simulink library "Battery"  (R2015a)
settings: Solver=ode45  StartTime=0.0  StopTime=10.0  RelTol=1e-3
undefined symbols (not defined in the file): Battery, Env, magnitude
libraries: fl_lib x10, nesl_utility x5
settings Model: Creator=tbria  LastModifiedBy=BRIAN

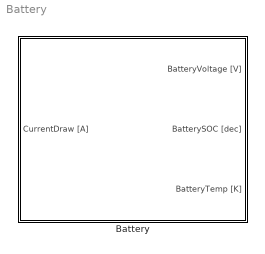
== system Battery ==
  Battery : Subsystem

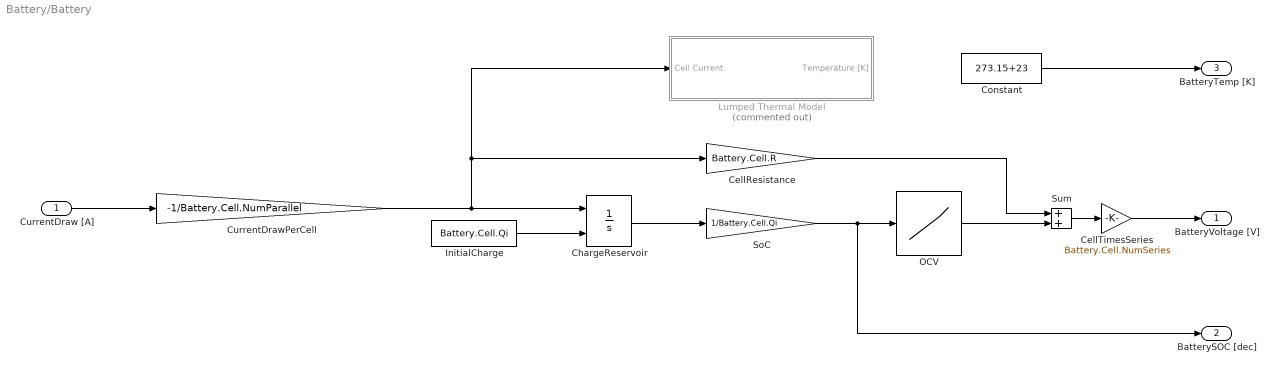
== system Battery/Battery ==
  CurrentDraw [A] : Inport
  CellResistance : Gain  Gain=Battery.Cell.R
  CellTimesSeries : Gain  Gain=Battery.Cell.NumSeries
  ChargeReservoir : Integrator  InitialConditionSource=external
  Constant : Constant  Value=273.15+23
  CurrentDrawPerCell : Gain  Gain=-1/Battery.Cell.NumParallel
  InitialCharge : Constant  Value=Battery.Cell.Qi
  Lumped Thermal Model : Subsystem  Commented=on
  OCV : Lookup_n-D  NumberOfTableDimensions=1  BreakpointsForDimension1=Battery.Cell.VoltOC.SoC  Table=Battery.Cell.VoltOC.Voltage  InternalRulePriority=Speed  RndMeth=Simplest  InputSameDT=on
  SoC : Gain  Gain=1/Battery.Cell.Qi
  Sum : Sum
  BatteryVoltage [V] : Outport
  BatterySOC [dec] : Outport  Port=2
  BatteryTemp [K] : Outport  Port=3
  wires:
  Constant/1 -> BatteryTemp [K]/1
  CurrentDraw [A]/1 -> CurrentDrawPerCell/1
  InitialCharge/1 -> ChargeReservoir/2
  ChargeReservoir/1 -> SoC/1
  SoC/1 -> OCV/1, BatterySOC [dec]/1
  CellTimesSeries/1 -> BatteryVoltage [V]/1
  CellResistance/1 -> Sum/1
  OCV/1 -> Sum/2
  Sum/1 -> CellTimesSeries/1
  CurrentDrawPerCell/1 -> Lumped Thermal Model/1(Cell Current), CellResistance/1, ChargeReservoir/1

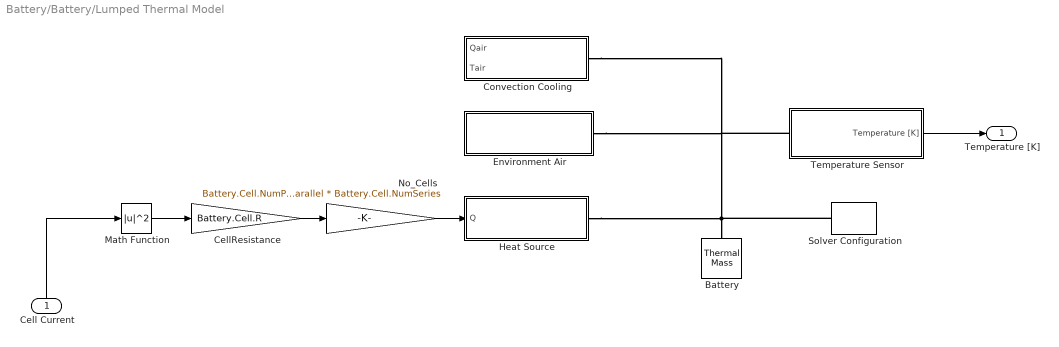
== system Battery/Battery/Lumped Thermal Model ==
  Cell Current : Inport
  Battery : fl_lib/Thermal/Thermal Elements/Thermal Mass  mass=Battery.Cell.m*Battery.Cell.NumParallel * Battery.Cell.NumSeries kg  sp_heat=Battery.Cell.c J/kg/K  Q_specify=off  Q_priority=High  Q=0 J/s  T_specify=off  T_priority=High  T=300 K
  CellResistance : Gain  Gain=Battery.Cell.R
  Convection Cooling : Subsystem
  Environment Air : Subsystem
  Heat Source : Subsystem
  Math Function : Math  Operator=magnitude^2  SaturateOnIntegerOverflow=on
  No_Cells : Gain  Gain=Battery.Cell.NumParallel * Battery.Cell.NumSeries
  Solver Configuration : nesl_utility/Solver Configuration  PhysicalDomain=network_engine_domain  SubClassName=solver  LeftPortType=input  RightPortType=generic  Accelerate=off  Tones=[]  Harmonics=[]  SimulateNoise=off  Profile=off  UseLocalSampling=off  EnableSwitchedLinearOptims=on  FrequencyDomain=off  UseCCode=off  RelTol=0.001  AbsTol=1e-06  MinStep=1e-09  ToWorkspace=off  RevertToSquareIcSolve=off  NumHomotopyIterations=100  DoDC=off  ResidualTolerance=1e-09  UseLocalSolver=off  LocalSolverChoice=NE_BACKWARD_EULER_ADVANCER  LocalSolverSampleTime=0.001  DoFixedCost=off  MaxNonlinIter=3  MaxModeIter=2  LinearAlgebra=Sparse  DelaysMemoryBudget=1024  AutomaticFiltering=on  FilteringTimeConstant=0.001
  Temperature Sensor : Subsystem
  Temperature [K] : Outport
  wires:
  Math Function/1 -> CellResistance/1
  CellResistance/1 -> No_Cells/1
  No_Cells/1 -> Heat Source/1(Q)
  Temperature Sensor/1(Temperature [K]) -> Temperature [K]/1
  Cell Current/1 -> Math Function/1
  connections:
  Heat Source/RConn1 -- Environment Air/RConn1 -- Temperature Sensor/LConn1 -- Convection Cooling/RConn1 -- Solver Configuration/RConn1 -- Battery/LConn1

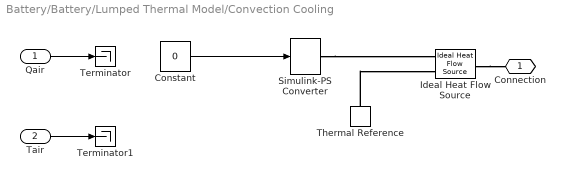
== system Battery/Battery/Lumped Thermal Model/Convection Cooling ==
  Qair : Inport
  Tair : Inport  Port=2
  Constant : Constant  Value=0
  Ideal Heat Flow Source : fl_lib/Thermal/Thermal Sources/Ideal Heat Flow Source
  Simulink-PS Converter : nesl_utility/Simulink-PS Converter  PhysicalDomain=network_engine_domain  SubClassName=ps_input  LeftPortType=input  RightPortType=output  PseudoPeriodic=off  Frequencies=[]  NoiseDistribution=none  NoiseParameters=[]  Unit=1  AffineConversion=off  InputFiltering=off  SimscapeFilterOrder=1  InputFilterTimeConstant=0.001  UdotUserProvided=1
  Terminator : Terminator
  Terminator1 : Terminator
  Thermal Reference : fl_lib/Thermal/Thermal Elements/Thermal Reference
  Connection : PMIOPort  Port=1  Side=Right
  wires:
  Tair/1 -> Terminator1/1
  Qair/1 -> Terminator/1
  Constant/1 -> Simulink-PS Converter/1
  connections:
  Simulink-PS Converter/RConn1 -- Ideal Heat Flow Source/RConn1
  Thermal Reference/LConn1 -- Ideal Heat Flow Source/RConn2
  Ideal Heat Flow Source/LConn1 -- Connection/RConn1

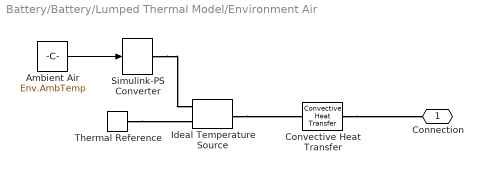
== system Battery/Battery/Lumped Thermal Model/Environment Air ==
  Ambient Air : Constant  Value=Env.AmbTemp
  Convective Heat Transfer : fl_lib/Thermal/Thermal Elements/Convective Heat Transfer  area=Battery.SA m^2  heat_tr_coeff=Env.NaturalConvection.K W/(m^2 * K)  Q_specify=off  Q_priority=High  Q=0 J/s  T_specify=off  T_priority=High  T=0 K
  Ideal Temperature Source : fl_lib/Thermal/Thermal Sources/Ideal Temperature Source
  Simulink-PS Converter : nesl_utility/Simulink-PS Converter  PhysicalDomain=network_engine_domain  SubClassName=ps_input  LeftPortType=input  RightPortType=output  PseudoPeriodic=off  Frequencies=[]  NoiseDistribution=none  NoiseParameters=[]  Unit=1  AffineConversion=off  InputFiltering=off  SimscapeFilterOrder=1  InputFilterTimeConstant=0.001  UdotUserProvided=1
  Thermal Reference : fl_lib/Thermal/Thermal Elements/Thermal Reference
  Connection : PMIOPort  Port=1  Side=Right
  wires:
  Ambient Air/1 -> Simulink-PS Converter/1
  connections:
  Ideal Temperature Source/LConn1 -- Convective Heat Transfer/LConn1
  Simulink-PS Converter/RConn1 -- Ideal Temperature Source/RConn1
  Thermal Reference/LConn1 -- Ideal Temperature Source/RConn2
  Convective Heat Transfer/RConn1 -- Connection/RConn1

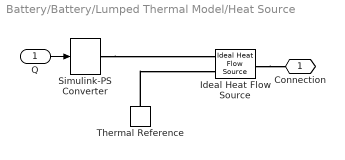
== system Battery/Battery/Lumped Thermal Model/Heat Source ==
  Q : Inport
  Ideal Heat Flow Source : fl_lib/Thermal/Thermal Sources/Ideal Heat Flow Source
  Simulink-PS Converter : nesl_utility/Simulink-PS Converter  PhysicalDomain=network_engine_domain  SubClassName=ps_input  LeftPortType=input  RightPortType=output  PseudoPeriodic=off  Frequencies=[]  NoiseDistribution=none  NoiseParameters=[]  Unit=1  AffineConversion=off  InputFiltering=off  SimscapeFilterOrder=1  InputFilterTimeConstant=0.001  UdotUserProvided=1
  Thermal Reference : fl_lib/Thermal/Thermal Elements/Thermal Reference
  Connection : PMIOPort  Port=1  Side=Right
  wires:
  Q/1 -> Simulink-PS Converter/1
  connections:
  Simulink-PS Converter/RConn1 -- Ideal Heat Flow Source/RConn1
  Thermal Reference/LConn1 -- Ideal Heat Flow Source/RConn2
  Ideal Heat Flow Source/LConn1 -- Connection/RConn1

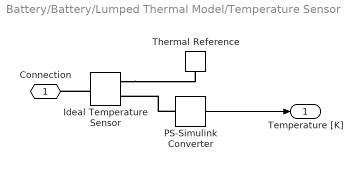
== system Battery/Battery/Lumped Thermal Model/Temperature Sensor ==
  Ideal Temperature Sensor : fl_lib/Thermal/Thermal Sensors/Ideal Temperature Sensor
  PS-Simulink Converter : nesl_utility/PS-Simulink Converter  PhysicalDomain=network_engine_domain  SubClassName=ps_output  LeftPortType=input  RightPortType=output  PseudoPeriodic=off  Frequencies=[]  Unit=1  AffineConversion=off
  Thermal Reference : fl_lib/Thermal/Thermal Elements/Thermal Reference
  Connection : PMIOPort  Port=1  Side=Left
  Temperature [K] : Outport
  wires:
  PS-Simulink Converter/1 -> Temperature [K]/1
  connections:
  Ideal Temperature Sensor/LConn1 -- Connection/RConn1
  PS-Simulink Converter/LConn1 -- Ideal Temperature Sensor/RConn2
  Ideal Temperature Sensor/RConn1 -- Thermal Reference/LConn1
